simulink model "dtc_gpc_temperatura_sim"  (R2020a)
settings: Solver=VariableStepAuto  StartTime=0.0  StopTime=tsim  MaxStep=0.01  RelTol=1e-3
values from neighbouring files (symbols this model uses):
  amppert = 0.05    [dtc_gpc_temperatura.m]
  amppert2 = 0    [dtc_gpc_temperatura.m]
  ampref = 0.5    [dtc_gpc_temperatura.m]
  Fdtc = Ftemp    [dtc_gpc_temperatura.m]
  Fgpc = Ftemp    [dtc_gpc_temperatura.m]
  Hdtc = cell2mat(H)    [dtc_gpc_temperatura.m]
  Hgpc = cell2mat(H)    [dtc_gpc_temperatura.m]
  Kdtc1 = [Kdtc1; Kdtc(sum(Nu(1:i-1))+1,:)]    [dtc_gpc_temperatura.m]
  Kgpc1 = [Kgpc1; Kgpc(sum(Nu(1:i-1))+1,:)]    [dtc_gpc_temperatura.m]
  tpert = 20    [dtc_gpc_temperatura.m]
  tpert2 = 0    [dtc_gpc_temperatura.m]
  tref = 2    [dtc_gpc_temperatura.m]
  Ts = 0.2    [dtc_gpc_temperatura.m]
  zr_dtc = blkdiag(zr_dtc,ones(Ny(i),1))    [dtc_gpc_temperatura.m]
  zr_gpc = blkdiag(zr_gpc,ones(Ny(i),1))    [dtc_gpc_temperatura.m]
libraries: cstblocks x8
settings Model: Creator=treezao  LastModifiedBy=treezao

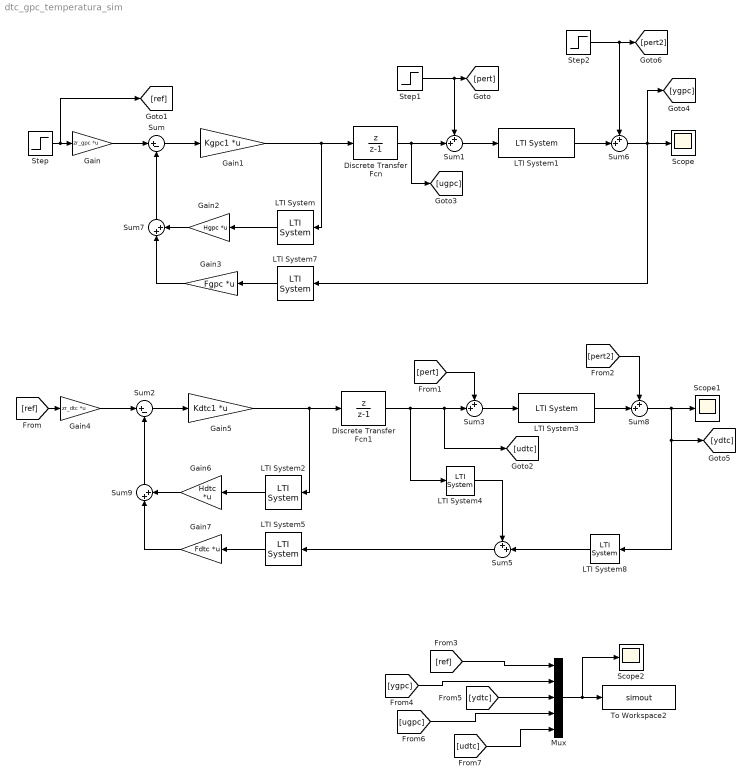
== system dtc_gpc_temperatura_sim ==
  Discrete Transfer Fcn : DiscreteTransferFcn  Numerator=[1 0]  Denominator=[1 -1]  SampleTime=Ts
  Discrete Transfer Fcn1 : DiscreteTransferFcn  Numerator=[1 0]  Denominator=[1 -1]  SampleTime=Ts
  Gain : Gain  Gain=zr_gpc  Multiplication=Matrix(K*u)
  Gain1 : Gain  Gain=Kgpc1  Multiplication=Matrix(K*u)
  Gain2 : Gain  Gain=Hgpc  Multiplication=Matrix(K*u)
  Gain3 : Gain  Gain=Fgpc  Multiplication=Matrix(K*u)
  Gain4 : Gain  Gain=zr_dtc  Multiplication=Matrix(K*u)
  Gain5 : Gain  Gain=Kdtc1  Multiplication=Matrix(K*u)
  Gain6 : Gain  Gain=Hdtc  Multiplication=Matrix(K*u)
  Gain7 : Gain  Gain=Fdtc  Multiplication=Matrix(K*u)
  LTI System : cstblocks/LTI System  sys=zu_gpc  IC=[]
  LTI System1 : cstblocks/LTI System  sys=P  IC=[]
  LTI System2 : cstblocks/LTI System  sys=zu_dtc  IC=[]
  LTI System3 : cstblocks/LTI System  sys=P  IC=[]
  LTI System4 : cstblocks/LTI System  sys=S  IC=[]
  LTI System5 : cstblocks/LTI System  sys=zy_dtc  IC=[]
  LTI System7 : cstblocks/LTI System  sys=zy_gpc  IC=[]
  LTI System8 : cstblocks/LTI System  sys=Fe  IC=[]
  Mux : Mux  Inputs=5
  Scope : Scope
  Scope1 : Scope
  Scope2 : Scope
  Step : Step  Time=tref  After=ampref  SampleTime=0
  Step1 : Step  Time=tpert  After=amppert  SampleTime=0
  Step2 : Step  Time=tpert2  After=amppert2  SampleTime=0
  Sum : Sum  Inputs=|+-
  Sum{1,3,5..6,8} (5 alike) : Sum  Inputs=++|
  Sum2 : Sum  Inputs=|+-
  Sum7 : Sum  Inputs=|++
  Sum9 : Sum  Inputs=|++
  To Workspace2 : ToWorkspace  VariableName=simout  SampleTime=-1
  wires:
  Step/1 -> [ref], Gain/1
  Sum/1 -> Gain1/1
  Gain1/1 -> LTI System/1, Discrete Transfer Fcn/1
  Step1/1 -> Sum1/1, [pert]
  Sum1/1 -> LTI System1/1
  Discrete Transfer Fcn1/1 -> [udtc], Sum3/2, LTI System4/1
  Sum3/1 -> LTI System3/1
  [pert] -> Sum3/1
  LTI System4/1 -> Sum5/1
  Sum8/1 -> LTI System8/1, [ydtc], Scope1/1
  Mux/1 -> Scope2/1, To Workspace2/1
  [ref] -> Mux/1
  [ygpc] -> Mux/2
  [ydtc] -> Mux/3
  [ugpc] -> Mux/4
  [udtc] -> Mux/5
  Step2/1 -> Sum6/1, [pert2]
  LTI System1/1 -> Sum6/2
  Sum6/1 -> LTI System7/1, [ygpc], Scope/1
  Gain/1 -> Sum/1
  Discrete Transfer Fcn/1 -> [ugpc], Sum1/2
  Sum7/1 -> Sum/2
  Gain2/1 -> Sum7/2
  LTI System/1 -> Gain2/1
  Gain3/1 -> Sum7/1
  LTI System7/1 -> Gain3/1
  LTI System3/1 -> Sum8/2
  [pert2] -> Sum8/1
  LTI System8/1 -> Sum5/2
  Gain6/1 -> Sum9/2
  LTI System5/1 -> Gain7/1
  LTI System2/1 -> Gain6/1
  Gain7/1 -> Sum9/1
  [ref] -> Gain4/1
  Gain5/1 -> LTI System2/1, Discrete Transfer Fcn1/1
  Gain4/1 -> Sum2/1
  Sum9/1 -> Sum2/2
  Sum2/1 -> Gain5/1
  Sum5/1 -> LTI System5/1
